simulink model "Prac6_Ejercicio"  (R2024b)
settings: Solver=FixedStepAuto  StartTime=0.0  StopTime=50  FixedStep=0.01  RelTol=1e-3
settings Model: Creator=PROBOOK  LastModifiedBy=PROBOOK

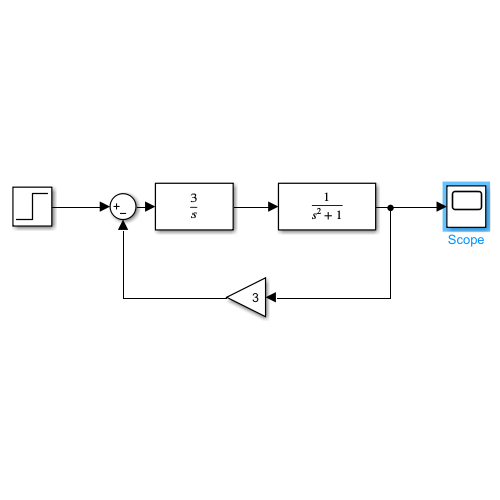
[thumbnail: Simulink's stored preview of the top-level diagram]
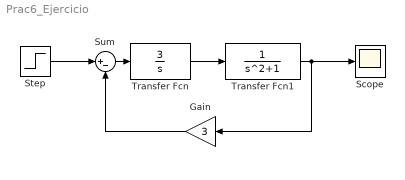
== system Prac6_Ejercicio ==
  Gain : Gain  Gain=3
  Scope : Scope
  Step : Step  Time=0  SampleTime=0
  Sum : Sum  Inputs=|+-
  Transfer Fcn : TransferFcn  Numerator=[3]  Denominator=[1 0]
  Transfer Fcn1 : TransferFcn  Denominator=[1 0 1]
  wires:
  Sum/1 -> Transfer Fcn/1
  Transfer Fcn1/1 -> Gain/1, Scope/1
  Gain/1 -> Sum/2
  Step/1 -> Sum/1
  Transfer Fcn/1 -> Transfer Fcn1/1
